simulink model "MCU_Input"  (R2022b)
settings: Solver=FixedStepDiscrete  StartTime=0.0  StopTime=10.0  FixedStep=1e-4  RelTol=1e-3
values from neighbouring files (symbols this model uses):
  C_ADC_Acc1Offset_i32 = 0.0    [MCU_Input_Sldd.sldd]    (also in MCU_Input_Sldd_objects.m = myPackage.Parameter)
  C_ADC_BrakeOffset_i32 = 0.0    [MCU_Input_Sldd.sldd]    (also in MCU_Input_Sldd_objects.m = myPackage.Parameter)
  C_ADC_HSTempGain_f32 = 0.0    [MCU_Input_Sldd.sldd]    (also in MCU_Input_Sldd_objects.m = myPackage.Parameter)
  C_ADC_HSTempOffset_i32 = 0.0    [MCU_Input_Sldd.sldd]    (also in MCU_Input_Sldd_objects.m = myPackage.Parameter)
  C_ADC_IdcOffset_i32 = 0.0    [MCU_Input_Sldd.sldd]    (also in MCU_Input_Sldd_objects.m = myPackage.Parameter)
  C_ADC_IGBTTable_i16 = 0.0    [MCU_Input_Sldd.sldd]    (also in MCU_Input_Sldd_objects.m = myPackage.Parameter)
  C_ADC_IGBTTempGain_f32 = 0.0    [MCU_Input_Sldd.sldd]    (also in MCU_Input_Sldd_objects.m = myPackage.Parameter)
  C_ADC_IGBTTempOffset_i32 = 0.0    [MCU_Input_Sldd.sldd]    (also in MCU_Input_Sldd_objects.m = myPackage.Parameter)
  C_ADC_MotorTemp1Gain_f32 = 0.0    [MCU_Input_Sldd.sldd]    (also in MCU_Input_Sldd_objects.m = myPackage.Parameter)
  C_ADC_MotorTemp1Offset_i32 = 0.0    [MCU_Input_Sldd.sldd]    (also in MCU_Input_Sldd_objects.m = myPackage.Parameter)
  C_ADC_MotorTempTable_i16 = 0.0    [MCU_Input_Sldd.sldd]    (also in MCU_Input_Sldd_objects.m = myPackage.Parameter)
  C_ADC_P12VOffset_i32 = 0.0    [MCU_Input_Sldd.sldd]    (also in MCU_Input_Sldd_objects.m = myPackage.Parameter)
  C_ADC_P15VOffset_i32 = 0.0    [MCU_Input_Sldd.sldd]    (also in MCU_Input_Sldd_objects.m = myPackage.Parameter)
  C_ADC_P5VOffset_i32 = 0.0    [MCU_Input_Sldd.sldd]    (also in MCU_Input_Sldd_objects.m = myPackage.Parameter)
  C_DCCurrent_DrvCoeff_f32 = 0.0    [MCU_Input_Sldd.sldd]    (also in MCU_Input_Sldd_objects.m = myPackage.Parameter)
  C_DCCurrent_GenCoeff_f32 = 0.0    [MCU_Input_Sldd.sldd]    (also in MCU_Input_Sldd_objects.m = myPackage.Parameter)
  C_Encoder_CurrentAdder_f32 = 0.0    [MCU_Input_Sldd.sldd]    (also in MCU_Input_Sldd_objects.m = myPackage.Parameter)
  C_Encoder_WaitTime_f32 = 0.0    [MCU_Input_Sldd.sldd]    (also in MCU_Input_Sldd_objects.m = myPackage.Parameter)
  C_Input_EncErr_u8 = 0.0    [MCU_Input_Sldd.sldd]    (also in MCU_Input_Sldd_objects.m = myPackage.Parameter)
  C_Rotate_RotateBits_u8 = 0.0    [MCU_Input_Sldd.sldd]    (also in MCU_Input_Sldd_objects.m = myPackage.Parameter)
  C_Rotate_SetAngle_u16 = 0.0    [MCU_Input_Sldd.sldd]    (also in MCU_Input_Sldd_objects.m = myPackage.Parameter)
  C_Rotate_SetAngleFlg_u8 = 0.0    [MCU_Input_Sldd.sldd]    (also in MCU_Input_Sldd_objects.m = myPackage.Parameter)
  C_SelfCheck_AvgCntSet_u16 = 0.0    [MCU_Input_Sldd.sldd]    (also in MCU_Input_Sldd_objects.m = myPackage.Parameter)
  C_SelfCheck_DelayTimeSet_u16 = 0.0    [MCU_Input_Sldd.sldd]    (also in MCU_Input_Sldd_objects.m = myPackage.Parameter)
  C_SelfCheck_IaoffsetDownLimt_u16 = 0.0    [MCU_Input_Sldd.sldd]    (also in MCU_Input_Sldd_objects.m = myPackage.Parameter)
  C_SelfCheck_IaoffsetUpLimt_u16 = 0.0    [MCU_Input_Sldd.sldd]    (also in MCU_Input_Sldd_objects.m = myPackage.Parameter)
  C_SelfCheck_IboffsetDownLimt_u16 = 0.0    [MCU_Input_Sldd.sldd]    (also in MCU_Input_Sldd_objects.m = myPackage.Parameter)
  C_SelfCheck_IboffsetUpLimt_u16 = 0.0    [MCU_Input_Sldd.sldd]    (also in MCU_Input_Sldd_objects.m = myPackage.Parameter)
  C_SelfCheck_IcoffsetDownLimt_u16 = 0.0    [MCU_Input_Sldd.sldd]    (also in MCU_Input_Sldd_objects.m = myPackage.Parameter)
  C_SelfCheck_IcoffsetUpLimt_u16 = 0.0    [MCU_Input_Sldd.sldd]    (also in MCU_Input_Sldd_objects.m = myPackage.Parameter)
  C_SelfCheck_OffsetUnCal_u8 = 0.0    [MCU_Input_Sldd.sldd]    (also in MCU_Input_Sldd_objects.m = myPackage.Parameter)
undefined symbols (not defined in the file or in its folder): AB_SAMPLE, ABC_SAMPLE, AC_SAMPLE, ANALOG, BC_SAMPLE, cAgeingMode, cParaRecogMode, cVvvfOpenMode, ParamCfg_AdAcc1K_u16, ParamCfg_AdBrakeK_u16, ParamCfg_AdIaK_u16, ParamCfg_AdIbK_u16, ParamCfg_AdIcK_u16, ParamCfg_AdKeyK_u16, ParamCfg_AdP12vK_u16, ParamCfg_AdP15vK_u16, ParamCfg_AdP5vK_u16, ParamCfg_AdUdcK_u16, ParamCfg_AdVonK_u16, ParamCfg_Avgcnt_u16, ParamCfg_BaseCur_u16, ParamCfg_BaseUdc_u16, ParamCfg_CommandSource_u16, ParamCfg_MaxSpeed_u16, ParamCfg_MotorNp_u16, ParamCfg_PosInit_u16, ParamCfg_PowerMax_u16, ParamCfg_PwmFreqLow_u16, ParamCfg_RotateDir_u16, ParamCfg_RotateNp_u16, ParamCfg_SampleMode_u16, ParamCfg_SensorSpeed_u16, ParamCfg_SmoPllKi_u16, ParamCfg_SmoPllKp_u16, ParamCfg_Stage_u16, ParamCfg_ThetaGain_u16, ParamCfg_UdcDefValue_u16, POWER_ON, STANDBY
libraries: simulink x41, YS_UserDefined_Library x4
(part 1 of 5)
settings Model: DataDictionary=MCU_Input_Sldd.sldd  Creator=ZYH  LastModifiedBy=ZYH
settings OptimizationCC: DefaultParameterBehavior=Inlined  EnhancedBackFolding=on  PassReuseOutputArgsAs=Individual arguments  OptimizeBlockOrder=speed  DifferentSizesBufferReuse=on  OptimizationCustomize=off  EfficientTunableParamExpr=on
settings DebuggingCC: ParameterTunabilityLossMsg=error
settings SFSimCC: MATLABDynamicMemAlloc=off
settings RTWCC: Description=Embedded Coder  SystemTargetFile=ert.tlc  GenCodeOnly=on  TemplateMakefile=ert_default_tmf
settings CodeAppCC: ForceParamTrailComments=on  IgnoreCustomStorageClasses=off  OperatorAnnotations=on  SimulinkDataObjDesc=on  SFDataObjDesc=on  InsertBlockDesc=on
settings ERTTargetCC: TargetLangStandard=C99 (ISO)  GenerateSampleERTMain=on  InlinedParameterPlacement=NonHierarchical  ERTCustomFileTemplate=example_file_process.tlc

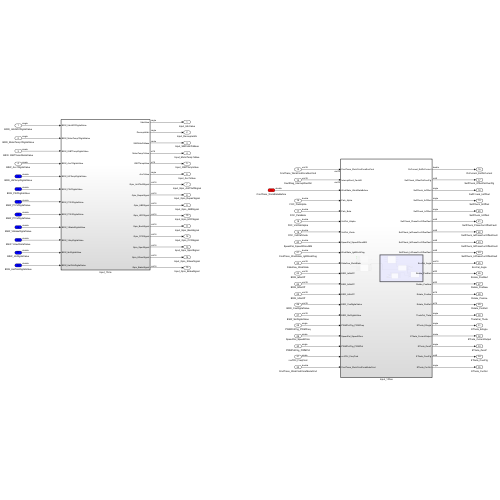
[thumbnail: Simulink's stored preview of the top-level diagram]
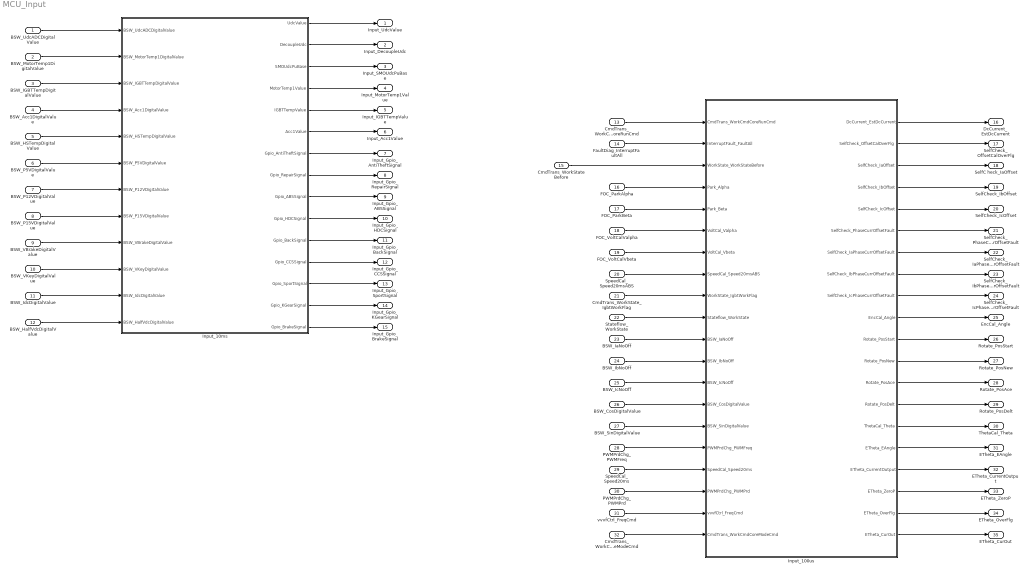
== system MCU_Input ==
  BSW_UdcADCDigitalValue : Inport
  BSW_MotorTemp1DigitalValue : Inport  Port=2
  BSW_IGBTTempDigitalValue : Inport  Port=3
  BSW_Acc1DigitalValue : Inport  Port=4
  BSW_HSTempDigitalValue : Inport  Port=5
  BSW_P5VDigitalValue : Inport  Port=6
  BSW_P12VDigitalValue : Inport  Port=7
  BSW_P15VDigitalValue : Inport  Port=8
  BSW_VBrakeDigitalValue : Inport  Port=9
  BSW_VKeyDigitalValue : Inport  Port=10
  BSW_IdcDigitalValue : Inport  Port=11
  BSW_HalfVdcDigitalValue : Inport  Port=12
  CmdTrans_WorkCmdCoreRunCmd : Inport  Port=13
  FaultDiag_InterruptFaultAll : Inport  Port=14
  CmdTrans_WorkStateBefore : Inport  Port=15
  FOC_ParkAlpha : Inport  Port=16
  FOC_ParkBeta : Inport  Port=17
  FOC_VoltCalValpha : Inport  Port=18
  FOC_VoltCalVbeta : Inport  Port=19
  SpeedCal_Speed20msABS : Inport  Port=20
  CmdTrans_WorkState_IgbtWorkFlag : Inport  Port=21
  Stateflow_WorkState : Inport  Port=22
  BSW_IaNoOff : Inport  Port=23
  BSW_IbNoOff : Inport  Port=24
  BSW_IcNoOff : Inport  Port=25
  BSW_CosDigitalValue : Inport  Port=26
  BSW_SinDigitalValue : Inport  Port=27
  PWMPrdChg_PWMFreq : Inport  Port=28
  SpeedCal_Speed20ms : Inport  Port=29
  PWMPrdChg_PWMPrd : Inport  Port=30
  vvvfCtrl_FreqCmd : Inport  Port=31
  CmdTrans_WorkCmdCoreModeCmd : Inport  Port=32
  Input_100us : Subsystem  TreatAsAtomicUnit=on
  Input_10ms : Subsystem  TreatAsAtomicUnit=on
  Input_UdcValue : Outport
  Input_DecoupleUdc : Outport  Port=2
  Input_SMOUdcPuBase : Outport  Port=3
  Input_MotorTemp1Value : Outport  Port=4
  Input_IGBTTempValue : Outport  Port=5
  Input_Acc1Value : Outport  Port=6
  Input_Gpio_AntiTheftSignal : Outport  Port=7
  Input_Gpio_RepairSignal : Outport  Port=8
  Input_Gpio_ABSSignal : Outport  Port=9
  Input_Gpio_HDCSignal : Outport  Port=10
  Input_Gpio_BackSignal : Outport  Port=11
  Input_Gpio_CCSSignal : Outport  Port=12
  Input_Gpio_SportSignal : Outport  Port=13
  Input_Gpio_KGearSignal : Outport  Port=14
  Input_Gpio_BrakeSignal : Outport  Port=15
  DcCurrent_EstDcCurrent : Outport  Port=16
  SelfCheck_OffsetCalOverFlg : Outport  Port=17
  SelfC heck_IaOffset : Outport  Port=18
  SelfCheck_IbOffset : Outport  Port=19
  SelfCheck_IcOffset : Outport  Port=20
  SelfCheck_PhaseCurrOffsetFault : Outport  Port=21
  SelfCheck_IaPhaseCurrOffsetFault : Outport  Port=22
  SelfCheck_IbPhaseCurrOffsetFault : Outport  Port=23
  SelfCheck_IcPhaseCurrOffsetFault : Outport  Port=24
  EncCal_Angle : Outport  Port=25
  Rotate_PosStart : Outport  Port=26
  Rotate_PosNew : Outport  Port=27
  Rotate_PosAce : Outport  Port=28
  Rotate_PosDelt : Outport  Port=29
  ThetaCal_Theta : Outport  Port=30
  ETheta_EAngle : Outport  Port=31
  ETheta_CurrentOutput : Outport  Port=32
  ETheta_ZeroP : Outport  Port=33
  ETheta_OverFlg : Outport  Port=34
  ETheta_CurOut : Outport  Port=35
  wires:
  BSW_IdcDigitalValue/1 -> Input_10ms/11(BSW_IdcDigitalValue)
  BSW_VKeyDigitalValue/1 -> Input_10ms/10(BSW_VKeyDigitalValue)
  Input_10ms/1(UdcValue) -> Input_UdcValue/1
  BSW_VBrakeDigitalValue/1 -> Input_10ms/9(BSW_VBrakeDigitalValue)
  BSW_P15VDigitalValue/1 -> Input_10ms/8(BSW_P15VDigitalValue)
  BSW_HalfVdcDigitalValue/1 -> Input_10ms/12(BSW_HalfVdcDigitalValue)
  BSW_Acc1DigitalValue/1 -> Input_10ms/4(BSW_Acc1DigitalValue)
  Input_10ms/5(IGBTTempValue) -> Input_IGBTTempValue/1
  Input_10ms/3(SMOUdcPuBase) -> Input_SMOUdcPuBase/1
  BSW_HSTempDigitalValue/1 -> Input_10ms/5(BSW_HSTempDigitalValue)
  BSW_P5VDigitalValue/1 -> Input_10ms/6(BSW_P5VDigitalValue)
  Input_10ms/2(DecoupleUdc) -> Input_DecoupleUdc/1
  BSW_IGBTTempDigitalValue/1 -> Input_10ms/3(BSW_IGBTTempDigitalValue)
  BSW_MotorTemp1DigitalValue/1 -> Input_10ms/2(BSW_MotorTemp1DigitalValue)
  BSW_P12VDigitalValue/1 -> Input_10ms/7(BSW_P12VDigitalValue)
  Input_10ms/6(Acc1Value) -> Input_Acc1Value/1
  Input_10ms/4(MotorTemp1Value) -> Input_MotorTemp1Value/1
  Input_10ms/7(Gpio_AntiTheftSignal) -> Input_Gpio_AntiTheftSignal/1
  Input_10ms/8(Gpio_RepairSignal) -> Input_Gpio_RepairSignal/1
  Input_10ms/9(Gpio_ABSSignal) -> Input_Gpio_ABSSignal/1
  Input_10ms/10(Gpio_HDCSignal) -> Input_Gpio_HDCSignal/1
  Input_10ms/11(Gpio_BackSignal) -> Input_Gpio_BackSignal/1
  Input_10ms/12(Gpio_CCSSignal) -> Input_Gpio_CCSSignal/1
  Input_10ms/13(Gpio_SportSignal) -> Input_Gpio_SportSignal/1
  Input_10ms/14(Gpio_KGearSignal) -> Input_Gpio_KGearSignal/1
  Input_10ms/15(Gpio_BrakeSignal) -> Input_Gpio_BrakeSignal/1
  CmdTrans_WorkCmdCoreRunCmd/1 -> Input_100us/1(CmdTrans_WorkCmdCoreRunCmd)
  FaultDiag_InterruptFaultAll/1 -> Input_100us/2(InterruptFault_FaultAll)
  Input_100us/1(DcCurrent_EstDcCurrent) -> DcCurrent_EstDcCurrent/1
  CmdTrans_WorkStateBefore/1 -> Input_100us/3(WorkState_WorkStateBefore)
  FOC_ParkAlpha/1 -> Input_100us/4(Park_Alpha)
  FOC_ParkBeta/1 -> Input_100us/5(Park_Beta)
  FOC_VoltCalValpha/1 -> Input_100us/6(VoltCal_Valpha)
  FOC_VoltCalVbeta/1 -> Input_100us/7(VoltCal_Vbeta)
  SpeedCal_Speed20msABS/1 -> Input_100us/8(SpeedCal_Speed20msABS)
  Stateflow_WorkState/1 -> Input_100us/10(Stateflow_WorkState)
  BSW_IaNoOff/1 -> Input_100us/11(BSW_IaNoOff)
  BSW_IbNoOff/1 -> Input_100us/12(BSW_IbNoOff)
  CmdTrans_WorkState_IgbtWorkFlag/1 -> Input_100us/9(WorkState_IgbtWorkFlag)
  BSW_IcNoOff/1 -> Input_100us/13(BSW_IcNoOff)
  Input_100us/3(SelfCheck_IaOffset) -> SelfC heck_IaOffset/1
  Input_100us/2(SelfCheck_OffsetCalOverFlg) -> SelfCheck_OffsetCalOverFlg/1
  Input_100us/4(SelfCheck_IbOffset) -> SelfCheck_IbOffset/1
  Input_100us/5(SelfCheck_IcOffset) -> SelfCheck_IcOffset/1
  Input_100us/6(SelfCheck_PhaseCurrOffsetFault) -> SelfCheck_PhaseCurrOffsetFault/1
  Input_100us/7(SelfCheck_IaPhaseCurrOffsetFault) -> SelfCheck_IaPhaseCurrOffsetFault/1
  Input_100us/8(SelfCheck_IbPhaseCurrOffsetFault) -> SelfCheck_IbPhaseCurrOffsetFault/1
  Input_100us/9(SelfCheck_IcPhaseCurrOffsetFault) -> SelfCheck_IcPhaseCurrOffsetFault/1
  BSW_UdcADCDigitalValue/1 -> Input_10ms/1(BSW_UdcADCDigitalValue)
  BSW_CosDigitalValue/1 -> Input_100us/14(BSW_CosDigitalValue)
  BSW_SinDigitalValue/1 -> Input_100us/15(BSW_SinDigitalValue)
  Input_100us/10(EncCal_Angle) -> EncCal_Angle/1
  Input_100us/11(Rotate_PosStart) -> Rotate_PosStart/1
  Input_100us/12(Rotate_PosNew) -> Rotate_PosNew/1
  Input_100us/13(Rotate_PosAce) -> Rotate_PosAce/1
  Input_100us/14(Rotate_PosDelt) -> Rotate_PosDelt/1
  SpeedCal_Speed20ms/1 -> Input_100us/17(SpeedCal_Speed20ms)
  PWMPrdChg_PWMPrd/1 -> Input_100us/18(PWMPrdChg_PWMPrd)
  vvvfCtrl_FreqCmd/1 -> Input_100us/19(vvvfCtrl_FreqCmd)
  CmdTrans_WorkCmdCoreModeCmd/1 -> Input_100us/20(CmdTrans_WorkCmdCoreModeCmd)
  Input_100us/15(ThetaCal_Theta) -> ThetaCal_Theta/1
  Input_100us/16(ETheta_EAngle) -> ETheta_EAngle/1
  Input_100us/17(ETheta_CurrentOutput) -> ETheta_CurrentOutput/1
  Input_100us/18(ETheta_ZeroP) -> ETheta_ZeroP/1
  Input_100us/19(ETheta_OverFlg) -> ETheta_OverFlg/1
  Input_100us/20(ETheta_CurOut) -> ETheta_CurOut/1
  PWMPrdChg_PWMFreq/1 -> Input_100us/16(PWMPrdChg_PWMFreq)

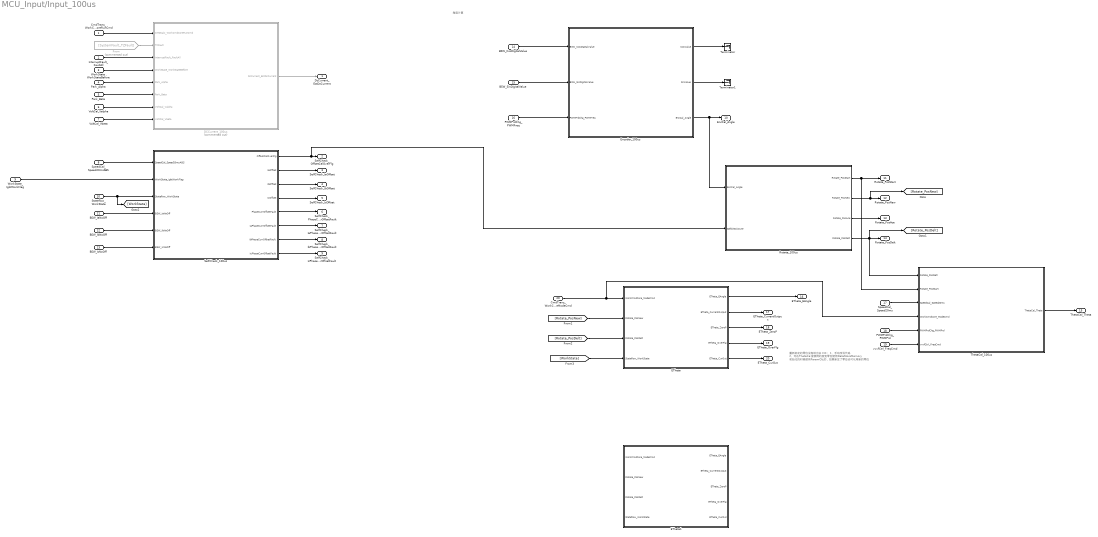
== system MCU_Input/Input_100us ==
  note: 重新标定的零位没有给出去
      | FIX：
      | 1、手动改写代码
      | 2、对在ThetaCal里使用的旋变零位使用DataStoreMemory
      | 	初始化的时候使用ParamCfg的，如果新定了零位也可以用新的零位
  note: 角度计算
  CmdTrans_WorkCmdCoreRunCmd : Inport  OutDataTypeStr=uint16
  InterruptFault_FaultAll : Inport  Port=2  OutDataTypeStr=uint16
  WorkState_WorkStateBefore : Inport  Port=3
  Park_Alpha : Inport  Port=4
  Park_Beta : Inport  Port=5
  VoltCal_Valpha : Inport  Port=6
  VoltCal_Vbeta : Inport  Port=7
  SpeedCal_Speed20msABS : Inport  Port=8
  WorkState_IgbtWorkFlag : Inport  Port=9
  Stateflow_WorkState : Inport  Port=10
  BSW_IaNoOff : Inport  Port=11
  BSW_IbNoOff : Inport  Port=12
  BSW_IcNoOff : Inport  Port=13
  BSW_CosDigitalValue : Inport  Port=14
  BSW_SinDigitalValue : Inport  Port=15
  PWMPrdChg_PWMFreq : Inport  Port=16
  SpeedCal_Speed20ms : Inport  Port=17
  PWMPrdChg_PWMPrd : Inport  Port=18
  vvvfCtrl_FreqCmd : Inport  Port=19
  CmdTrans_WorkCmdCoreModeCmd : Inport  Port=20
  DCCurrent_100us : Subsystem  Commented=on  TreatAsAtomicUnit=on
      settings: RTWSystemCode=Nonreusable function
  ETheta : Subsystem
  ETheta1 : Subsystem
  Encoder_100us : Subsystem  TreatAsAtomicUnit=on
      settings: RTWSystemCode=Nonreusable function
  From : From  Commented=on  GotoTag=SystemFault_TZFault
  Rotate_100us : Subsystem  TreatAsAtomicUnit=on
      settings: RTWSystemCode=Nonreusable function
  SelfCheck_100us : Subsystem  TreatAsAtomicUnit=on
      settings: RTWSystemCode=Nonreusable function
  Terminator : Terminator
  Terminator1 : Terminator
  ThetaCal_100us : Subsystem
  DcCurrent_EstDcCurrent : Outport
  SelfCheck_OffsetCalOverFlg : Outport  Port=2
  SelfCheck_IaOffset : Outport  Port=3
  SelfCheck_IbOffset : Outport  Port=4
  SelfCheck_IcOffset : Outport  Port=5
  SelfCheck_PhaseCurrOffsetFault : Outport  Port=6
  SelfCheck_IaPhaseCurrOffsetFault : Outport  Port=7
  SelfCheck_IbPhaseCurrOffsetFault : Outport  Port=8
  SelfCheck_IcPhaseCurrOffsetFault : Outport  Port=9
  EncCal_Angle : Outport  Port=10
  Rotate_PosStart : Outport  Port=11
  Rotate_PosNew : Outport  Port=12
  Rotate_PosAce : Outport  Port=13
  Rotate_PosDelt : Outport  Port=14
  ThetaCal_Theta : Outport  Port=15
  ETheta_EAngle : Outport  Port=16
  ETheta_CurrentOutput : Outport  Port=17
  ETheta_ZeroP : Outport  Port=18
  ETheta_OverFlg : Outport  Port=19
  ETheta_CurOut : Outport  Port=20
  wires:
  CmdTrans_WorkCmdCoreRunCmd/1 -> DCCurrent_100us/1(CMDCalc_WorkCmdCoreRunCmd)
  From/1 -> DCCurrent_100us/2(TZFault)
  InterruptFault_FaultAll/1 -> DCCurrent_100us/3(InterruptFault_FaultAll)
  DCCurrent_100us/1(DcCurrent_EstDcCurrent) -> DcCurrent_EstDcCurrent/1
  WorkState_WorkStateBefore/1 -> DCCurrent_100us/4(WorkState_WorkStateBefore)
  Park_Alpha/1 -> DCCurrent_100us/5(Park_Alpha)
  Park_Beta/1 -> DCCurrent_100us/6(Park_Beta)
  VoltCal_Valpha/1 -> DCCurrent_100us/7(VoltCal_Valpha)
  VoltCal_Vbeta/1 -> DCCurrent_100us/8(VoltCal_Vbeta)
  SpeedCal_Speed20msABS/1 -> SelfCheck_100us/1(SpeedCal_Speed20msABS)
  WorkState_IgbtWorkFlag/1 -> SelfCheck_100us/2(WorkState_IgbtWorkFlag)
  Stateflow_WorkState/1 -> [WorkState], SelfCheck_100us/3(Stateflow_WorkState)
  BSW_IaNoOff/1 -> SelfCheck_100us/4(BSW_IaNoOff)
  BSW_IbNoOff/1 -> SelfCheck_100us/5(BSW_IbNoOff)
  BSW_IcNoOff/1 -> SelfCheck_100us/6(BSW_IcNoOff)
  SelfCheck_100us/1(OffsetCalOverFlg) -> Rotate_100us/2(SelfCheckOver), SelfCheck_OffsetCalOverFlg/1
  SelfCheck_100us/2(IaOffset) -> SelfCheck_IaOffset/1
  SelfCheck_100us/5(PhaseCurrOffsetFault) -> SelfCheck_PhaseCurrOffsetFault/1
  SelfCheck_100us/4(IcOffset) -> SelfCheck_IcOffset/1
  SelfCheck_100us/3(IbOffset) -> SelfCheck_IbOffset/1
  SelfCheck_100us/7(IbPhaseCurrOffsetFault) -> SelfCheck_IbPhaseCurrOffsetFault/1
  SelfCheck_100us/6(IaPhaseCurrOffsetFault) -> SelfCheck_IaPhaseCurrOffsetFault/1
  SelfCheck_100us/8(IcPhaseCurrOffsetFault) -> SelfCheck_IcPhaseCurrOffsetFault/1
  BSW_CosDigitalValue/1 -> Encoder_100us/1(BSW_CosDigitalValue)
  BSW_SinDigitalValue/1 -> Encoder_100us/2(BSW_SinDigitalValue)
  Encoder_100us/1(CosValue) -> Terminator/1
  Encoder_100us/2(SinValue) -> Terminator1/1
  Encoder_100us/3(EncCal_Angle) -> Rotate_100us/1(EncCal_Angle), EncCal_Angle/1
  Rotate_100us/1(Rotate_PosStart) -> ThetaCal_100us/2(Rotate_PosStart), Rotate_PosStart/1
  Rotate_100us/2(Rotate_PosNew) -> [Rotate_PosNew], Rotate_PosNew/1
  Rotate_100us/3(Rotate_PosAce) -> Rotate_PosAce/1
  Rotate_100us/4(Rotate_PosDelt) -> ThetaCal_100us/1(Rotate_PosDelt), [Rotate_PosDelt], Rotate_PosDelt/1
  SpeedCal_Speed20ms/1 -> ThetaCal_100us/3(SpeedCal_Speed20ms)
  ThetaCal_100us/1(ThetaCal_Theta) -> ThetaCal_Theta/1
  CmdTrans_WorkCmdCoreModeCmd/1 -> ThetaCal_100us/4(WorkCmdCore_ModeCmd), ETheta/1(WorkCmdCore_ModeCmd)
  PWMPrdChg_PWMPrd/1 -> ThetaCal_100us/5(PWMPrdChg_PWMPrd)
  vvvfCtrl_FreqCmd/1 -> ThetaCal_100us/6(vvvfCtrl_FreqCmd)
  [Rotate_PosNew] -> ETheta/2(Rotate_PosNew)
  [Rotate_PosDelt] -> ETheta/3(Rotate_PosDelt)
  ETheta/1(ETheta_EAngle) -> ETheta_EAngle/1
  ETheta/2(ETheta_CurrentOutput) -> ETheta_CurrentOutput/1
  ETheta/3(ETheta_ZeroP) -> ETheta_ZeroP/1
  ETheta/4(ETheta_OverFlg) -> ETheta_OverFlg/1
  ETheta/5(ETheta_CurOut) -> ETheta_CurOut/1
  PWMPrdChg_PWMFreq/1 -> Encoder_100us/3(PWMPrdChg_PWMFreq)
  [WorkState] -> ETheta/4(Stateflow_WorkState)

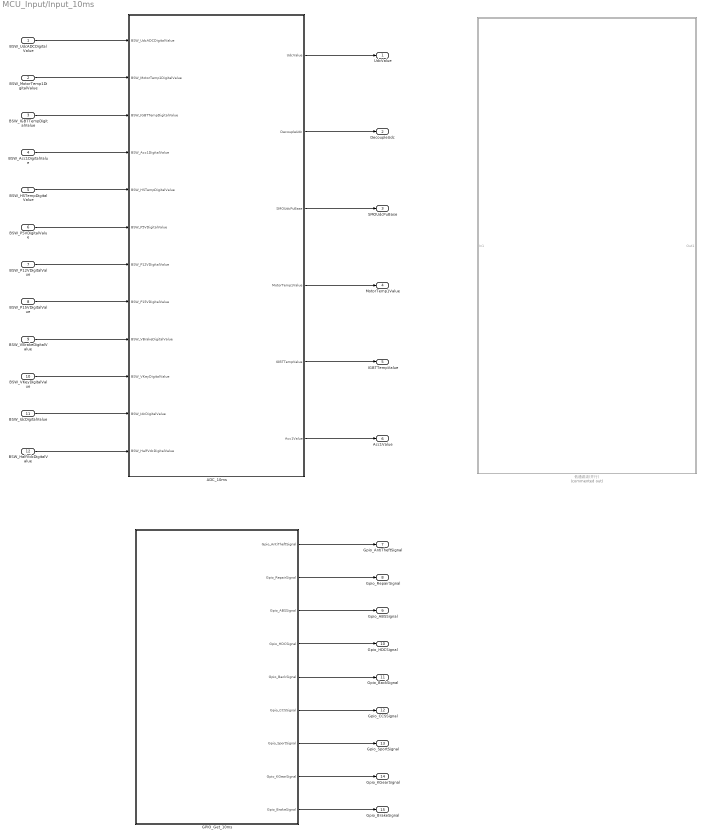
== system MCU_Input/Input_10ms ==
  BSW_UdcADCDigitalValue : Inport
  BSW_MotorTemp1DigitalValue : Inport  Port=2
  BSW_IGBTTempDigitalValue : Inport  Port=3
  BSW_Acc1DigitalValue : Inport  Port=4
  BSW_HSTempDigitalValue : Inport  Port=5
  BSW_P5VDigitalValue : Inport  Port=6
  BSW_P12VDigitalValue : Inport  Port=7
  BSW_P15VDigitalValue : Inport  Port=8
  BSW_VBrakeDigitalValue : Inport  Port=9
  BSW_VKeyDigitalValue : Inport  Port=10
  BSW_IdcDigitalValue : Inport  Port=11
  BSW_HalfVdcDigitalValue : Inport  Port=12
  ADC_10ms : Subsystem  TreatAsAtomicUnit=on
      settings: RTWSystemCode=Nonreusable function
  GPIO_Get_10ms : Subsystem  TreatAsAtomicUnit=on
      settings: RTWSystemCode=Nonreusable function
  低通滤波(并行) : Subsystem  Commented=on
  UdcValue : Outport
  DecoupleUdc : Outport  Port=2
  SMOUdcPuBase : Outport  Port=3
  MotorTemp1Value : Outport  Port=4
  IGBTTempValue : Outport  Port=5
  Acc1Value : Outport  Port=6
  Gpio_AntiTheftSignal : Outport  Port=7
  Gpio_RepairSignal : Outport  Port=8
  Gpio_ABSSignal : Outport  Port=9
  Gpio_HDCSignal : Outport  Port=10
  Gpio_BackSignal : Outport  Port=11
  Gpio_CCSSignal : Outport  Port=12
  Gpio_SportSignal : Outport  Port=13
  Gpio_KGearSignal : Outport  Port=14
  Gpio_BrakeSignal : Outport  Port=15
  wires:
  BSW_MotorTemp1DigitalValue/1 -> ADC_10ms/2(BSW_MotorTemp1DigitalValue)
  BSW_IGBTTempDigitalValue/1 -> ADC_10ms/3(BSW_IGBTTempDigitalValue)
  BSW_Acc1DigitalValue/1 -> ADC_10ms/4(BSW_Acc1DigitalValue)
  BSW_HSTempDigitalValue/1 -> ADC_10ms/5(BSW_HSTempDigitalValue)
  BSW_P5VDigitalValue/1 -> ADC_10ms/6(BSW_P5VDigitalValue)
  BSW_P12VDigitalValue/1 -> ADC_10ms/7(BSW_P12VDigitalValue)
  BSW_P15VDigitalValue/1 -> ADC_10ms/8(BSW_P15VDigitalValue)
  BSW_VBrakeDigitalValue/1 -> ADC_10ms/9(BSW_VBrakeDigitalValue)
  BSW_VKeyDigitalValue/1 -> ADC_10ms/10(BSW_VKeyDigitalValue)
  BSW_IdcDigitalValue/1 -> ADC_10ms/11(BSW_IdcDigitalValue)
  BSW_HalfVdcDigitalValue/1 -> ADC_10ms/12(BSW_HalfVdcDigitalValue)
  ADC_10ms/4(MotorTemp1Value) -> MotorTemp1Value/1
  ADC_10ms/3(SMOUdcPuBase) -> SMOUdcPuBase/1
  ADC_10ms/5(IGBTTempValue) -> IGBTTempValue/1
  ADC_10ms/2(DecoupleUdc) -> DecoupleUdc/1
  ADC_10ms/6(Acc1Value) -> Acc1Value/1
  ADC_10ms/1(UdcValue) -> UdcValue/1
  GPIO_Get_10ms/1(Gpio_AntiTheftSignal) -> Gpio_AntiTheftSignal/1
  GPIO_Get_10ms/2(Gpio_RepairSignal) -> Gpio_RepairSignal/1
  GPIO_Get_10ms/3(Gpio_ABSSignal) -> Gpio_ABSSignal/1
  GPIO_Get_10ms/4(Gpio_HDCSignal) -> Gpio_HDCSignal/1
  GPIO_Get_10ms/5(Gpio_BackSignal) -> Gpio_BackSignal/1
  GPIO_Get_10ms/6(Gpio_CCSSignal) -> Gpio_CCSSignal/1
  GPIO_Get_10ms/7(Gpio_SportSignal) -> Gpio_SportSignal/1
  GPIO_Get_10ms/8(Gpio_KGearSignal) -> Gpio_KGearSignal/1
  GPIO_Get_10ms/9(Gpio_BrakeSignal) -> Gpio_BrakeSignal/1
  BSW_UdcADCDigitalValue/1 -> ADC_10ms/1(BSW_UdcADCDigitalValue)

== system MCU_Input/Input_100us/DCCurrent_100us ==
  CMDCalc_WorkCmdCoreRunCmd : Inport
  TZFault : Inport  Port=2
  InterruptFault_FaultAll : Inport  Port=3
  WorkState_WorkStateBefore : Inport  Port=4
  Park_Alpha : Inport  Port=5
  Park_Beta : Inport  Port=6
  VoltCal_Valpha : Inport  Port=7
  VoltCal_Vbeta : Inport  Port=8
  Compare To Constant : simulink/Logic and Bit Operations/Compare To Constant  relop===  const=1  OutDataTypeStr=boolean
  Compare To Constant1 : simulink/Logic and Bit Operations/Compare To Constant  relop===  const=0  OutDataTypeStr=boolean
  Compare To Constant2 : simulink/Logic and Bit Operations/Compare To Constant  relop===  const=0  OutDataTypeStr=boolean
  DcCurrentCal : Subsystem  TreatAsAtomicUnit=on
  Logical Operator : Logic  Inputs=3  AllPortsSameDT=off  OutDataTypeStr=boolean
  DcCurrent_EstDcCurrent : Outport
  wires:
  CMDCalc_WorkCmdCoreRunCmd/1 -> Compare To Constant/1
  TZFault/1 -> Compare To Constant1/1
  InterruptFault_FaultAll/1 -> Compare To Constant2/1
  Compare To Constant1/1 -> Logical Operator/2
  Compare To Constant2/1 -> Logical Operator/3
  Compare To Constant/1 -> Logical Operator/1
  Logical Operator/1 -> DcCurrentCal/Enable
  DcCurrentCal/1(DcCurrent_EstDcCurrent) -> DcCurrent_EstDcCurrent/1
  WorkState_WorkStateBefore/1 -> DcCurrentCal/1(WorkState_WorkStateBefore)
  Park_Alpha/1 -> DcCurrentCal/2(Park_Alpha)
  Park_Beta/1 -> DcCurrentCal/3(Park_Beta)
  VoltCal_Valpha/1 -> DcCurrentCal/4(VoltCal_Valpha)
  VoltCal_Vbeta/1 -> DcCurrentCal/5(VoltCal_Vbeta)

== system MCU_Input/Input_100us/ETheta ==
  WorkCmdCore_ModeCmd : Inport
  Rotate_PosNew : Inport  Port=2
  Rotate_PosDelt : Inport  Port=3
  Stateflow_WorkState : Inport  Port=4
  Compare To Constant : simulink/Logic and Bit Operations/Compare To Constant  relop===  const=cParaRecogMode  OutDataTypeStr=boolean
  Compare To Constant1 : simulink/Logic and Bit Operations/Compare To Constant  relop===  const=STANDBY  OutDataTypeStr=boolean
  Constant : Constant  Value=0  OutDataTypeStr=single
  En : Subsystem
  Switch : Switch  Criteria=u2 ~= 0  SaturateOnIntegerOverflow=off  InputSameDT=off
  Switch1 : Switch  Criteria=u2 ~= 0  SaturateOnIntegerOverflow=off  InputSameDT=off
  ETheta_EAngle : Outport
  ETheta_CurrentOutput : Outport  Port=2
  ETheta_ZeroP : Outport  Port=3
  ETheta_OverFlg : Outport  Port=4
  ETheta_CurOut : Outport  Port=5
  wires:
  Rotate_PosNew/1 -> En/1(Rotate_PosNew)
  Rotate_PosDelt/1 -> En/2(Rotate_PosDelt)
  WorkCmdCore_ModeCmd/1 -> Compare To Constant/1
  Compare To Constant/1 -> En/Enable
  En/1(EAngle) -> Switch/3
  En/2(CurrentOutput) -> Switch1/3
  En/4(OverFlg) -> ?
  En/5(CurOut) -> ?
  Stateflow_WorkState/1 -> Compare To Constant1/1
  Compare To Constant1/1 -> Switch1/2, Switch/2
  Constant/1 -> Switch1/1, Switch/1
  Switch/1 -> ETheta_EAngle/1
  Switch1/1 -> ETheta_CurrentOutput/1
  En/3(ZeroP) -> ETheta_ZeroP/1

== system MCU_Input/Input_100us/ETheta1 ==
  WorkCmdCore_ModeCmd : Inport
  Rotate_PosNew : Inport  Port=2
  Rotate_PosDelt : Inport  Port=3
  Stateflow_WorkState : Inport  Port=4
  Compare To Constant : simulink/Logic and Bit Operations/Compare To Constant  relop===  const=cParaRecogMode  OutDataTypeStr=boolean
  Compare To Constant1 : simulink/Logic and Bit Operations/Compare To Constant  relop===  const=STANDBY  OutDataTypeStr=boolean
  En : Subsystem
  ETheta_EAngle : Outport
  ETheta_CurrentOutput : Outport  Port=2
  ETheta_ZeroP : Outport  Port=3
  ETheta_OverFlg : Outport  Port=4
  ETheta_CurOut : Outport  Port=5
  wires:
  Rotate_PosNew/1 -> En/2(Rotate_PosNew)
  Rotate_PosDelt/1 -> En/3(Rotate_PosDelt)
  WorkCmdCore_ModeCmd/1 -> Compare To Constant/1
  Compare To Constant/1 -> En/1(cParaRecogMode)
  Stateflow_WorkState/1 -> Compare To Constant1/1
  Compare To Constant1/1 -> En/4(Standby)
  En/3(ZeroP) -> ETheta_ZeroP/1
  En/1(EAngle) -> ETheta_EAngle/1
  En/2(CurrentOutput) -> ETheta_CurrentOutput/1
  En/4(OverFlg) -> ETheta_OverFlg/1
  En/5(CurOut) -> ETheta_CurOut/1

== system MCU_Input/Input_100us/Encoder_100us ==
  note: 源代码这里除了有感还有无感，才有了这个使能，模型现在只有有感，暂时屏蔽这个使能
  BSW_CosDigitalValue : Inport
  BSW_SinDigitalValue : Inport  Port=2
  PWMPrdChg_PWMFreq : Inport  Port=3
  Compare To Constant : simulink/Logic and Bit Operations/Compare To Constant  Commented=on  relop===  const=1  OutDataTypeStr=boolean
  Constant : Constant  Value=ParamCfg_Stage_u16
  Constant1 : Constant  Value=ParamCfg_Avgcnt_u16
  Constant2 : Constant  Commented=on  Value=ParamCfg_SensorSpeed_u16
  Encoder_100us : Subsystem
  CosValue : Outport
  SinValue : Outport  Port=2
  EncCal_Angle : Outport  Port=3
  wires:
  BSW_CosDigitalValue/1 -> Encoder_100us/3(CosDigitalValue)
  BSW_SinDigitalValue/1 -> Encoder_100us/4(SinDigitalValue)
  Encoder_100us/1(CosAverage) -> CosValue/1
  Encoder_100us/2(SinAverage) -> SinValue/1
  Constant/1 -> Encoder_100us/1(Calib_Stage)
  Constant1/1 -> Encoder_100us/2(AvgCnt)
  Encoder_100us/3(EncCal_Angle) -> EncCal_Angle/1
  PWMPrdChg_PWMFreq/1 -> Encoder_100us/5(PWMPrdChg_PWMFreq)
  Constant2/1 -> Compare To Constant/1

== system MCU_Input/Input_100us/Rotate_100us ==
  EncCal_Angle : Inport
  SelfCheckOver : Inport  Port=2
  RotateCalc : Subsystem
  Rotate_PosStart : Outport
  Rotate_PosNew : Outport  Port=2
  Rotate_PosAce : Outport  Port=3
  Rotate_PosDelt : Outport  Port=4
  wires:
  EncCal_Angle/1 -> RotateCalc/1(EncCal_Angle)
  RotateCalc/1(Rotate_PosStart) -> Rotate_PosStart/1
  RotateCalc/2(Rotate_PosNew) -> Rotate_PosNew/1
  RotateCalc/3(Rotate_PosAce) -> Rotate_PosAce/1
  RotateCalc/4(Rotate_PosDelt) -> Rotate_PosDelt/1
  SelfCheckOver/1 -> RotateCalc/2(SelfCheckOver)

== system MCU_Input/Input_100us/SelfCheck_100us ==
  note: 在standby状态下持续执行
      | 在poweron状态下只执行一次
  SpeedCal_Speed20msABS : Inport
  WorkState_IgbtWorkFlag : Inport  Port=2
  Stateflow_WorkState : Inport  Port=3  OutDataTypeStr=uint16
  BSW_IaNoOff : Inport  Port=4
  BSW_IbNoOff : Inport  Port=5
  BSW_IcNoOff : Inport  Port=6
  Compare To Constant : simulink/Logic and Bit Operations/Compare To Constant  relop===  const=POWER_ON  OutDataTypeStr=uint8
  Compare To Constant2 : simulink/Logic and Bit Operations/Compare To Constant  relop===  const=STANDBY  OutDataTypeStr=uint8
  Constant : Constant  Value=C_SelfCheck_DelayTimeSet_u16  OutDataTypeStr=uint16
  Constant1 : Constant  Value=C_SelfCheck_AvgCntSet_u16  OutDataTypeStr=uint16
  Constant4 : Constant  Value=ParamCfg_SampleMode_u16
  EnCal : Subsystem
  OffsetCal : Subsystem
      settings: RTWSystemCode=Inline
  OffsetCalOverFlg : Outport
  IaOffset : Outport  Port=2
  IbOffset : Outport  Port=3
  IcOffset : Outport  Port=4
  PhaseCurrOffsetFault : Outport  Port=5
  IaPhaseCurrOffsetFault : Outport  Port=6
  IbPhaseCurrOffsetFault : Outport  Port=7
  IcPhaseCurrOffsetFault : Outport  Port=8
  wires:
  Constant4/1 -> OffsetCal/3(ParamCfg_SampleMode)
  OffsetCal/4(IcOffset) -> IcOffset/1
  Compare To Constant2/1 -> OffsetCal/1(StandbyState), EnCal/3(StanbyState)
  Constant1/1 -> OffsetCal/8(AvgCntSet)
  Compare To Constant/1 -> OffsetCal/2(PoweronState), EnCal/4(PoweronState)
  OffsetCal/7(IbOffsetFault) -> IbPhaseCurrOffsetFault/1
  OffsetCal/1(OffsetCalOverFlg) -> [OffsetCalOverFlg], OffsetCalOverFlg/1
  OffsetCal/3(IbOffset) -> IbOffset/1
  BSW_IcNoOff/1 -> OffsetCal/6(BSW_IcNoOff)
  OffsetCal/5(PhaseCurrOffsetFault) -> PhaseCurrOffsetFault/1
  Stateflow_WorkState/1 -> Compare To Constant/1, Compare To Constant2/1
  Constant/1 -> OffsetCal/7(DelayTimeSet)
  OffsetCal/8(IcOffsetFault) -> IcPhaseCurrOffsetFault/1
  OffsetCal/2(IaOffset) -> IaOffset/1
  BSW_IbNoOff/1 -> OffsetCal/5(BSW_IbNoOff)
  OffsetCal/6(IaOffsetFault) -> IaPhaseCurrOffsetFault/1
  BSW_IaNoOff/1 -> OffsetCal/4(BSW_IaNoOff)
  SpeedCal_Speed20msABS/1 -> EnCal/1(SpeedCal_Speed20msABS)
  WorkState_IgbtWorkFlag/1 -> EnCal/2(WorkState_IgbtWorkFlag)
  EnCal/1(M_Selfcheck_EnFlg_u8) -> OffsetCal/Enable
  [OffsetCalOverFlg] -> EnCal/5(OffsetCalOverFlg)

== system MCU_Input/Input_100us/ThetaCal_100us ==
  Rotate_PosDelt : Inport
  Rotate_PosStart : Inport  Port=2
  SpeedCal_Speed20ms : Inport  Port=3
  WorkCmdCore_ModeCmd : Inport  Port=4
  PWMPrdChg_PWMPrd : Inport  Port=5
  vvvfCtrl_FreqCmd : Inport  Port=6
  Compare To Constant : simulink/Logic and Bit Operations/Compare To Constant  relop===  const=1  OutDataTypeStr=boolean
  Compare To Constant1 : simulink/Logic and Bit Operations/Compare To Constant  relop===  const=cVvvfOpenMode  OutDataTypeStr=boolean
  Compare To Constant2 : simulink/Logic and Bit Operations/Compare To Constant  relop===  const=cAgeingMode  OutDataTypeStr=boolean
  Compare To Constant3 : simulink/Logic and Bit Operations/Compare To Constant  relop=>  const=1  OutDataTypeStr=boolean
  Compare To Constant4 : simulink/Logic and Bit Operations/Compare To Constant  relop=<  const=0  OutDataTypeStr=boolean
  Constant : Constant  Value=ParamCfg_SensorSpeed_u16
  Constant4 : Constant  Value=0  OutDataTypeStr=single
  If : If  NumInputs=2  IfExpression=u1 == 1  ElseIfExpressions=u2==1
  If Action Subsystem : Subsystem  TreatAsAtomicUnit=on
  If Action Subsystem1 : Subsystem  TreatAsAtomicUnit=on
  If Action Subsystem2 : Subsystem  TreatAsAtomicUnit=on
  Logical Operator : Logic  Operator=OR  AllPortsSameDT=off  OutDataTypeStr=boolean
  Merge : Merge  Inputs=3
  Switch : Switch  Criteria=u2 ~= 0  SaturateOnIntegerOverflow=off  InputSameDT=off
  ThetaCal : Subsystem
  ThetaOffsetGain : Subsystem
  ThetaCal_Theta : Outport
  wires:
  Constant/1 -> ThetaOffsetGain/1(SpeedSensor), Compare To Constant/1
  Rotate_PosDelt/1 -> ThetaCal/1(Rotate_PosDelt)
  Rotate_PosStart/1 -> ThetaCal/2(Rotate_PosStart)
  SpeedCal_Speed20ms/1 -> ThetaOffsetGain/2(SpeedCal_Speed20ms)
  ThetaOffsetGain/1(PosCompensate) -> ThetaCal/3(PosCompensate)
  Compare To Constant/1 -> ThetaCal/Enable
  WorkCmdCore_ModeCmd/1 -> Compare To Constant2/1, Compare To Constant1/1
  Compare To Constant1/1 -> If/1
  Compare To Constant2/1 -> If/2
  If/1 -> If Action Subsystem/Action
  PWMPrdChg_PWMPrd/1 -> If Action Subsystem1/1(PWMPrdChg_PWMPrd), If Action Subsystem/1(PWMPrdChg_PWMPrd)
  vvvfCtrl_FreqCmd/1 -> If Action Subsystem1/2(vvvfCtrl_FreqCmd), If Action Subsystem/2(vvvfCtrl_FreqCmd)
  If/2 -> If Action Subsystem1/Action
  If/3 -> If Action Subsystem2/Action
  ThetaCal/1(POSTheta) -> If Action Subsystem2/1(POSTheta)
  If Action Subsystem/1(mTheta) -> Merge/1
  If Action Subsystem1/1(mTheta) -> Merge/2
  If Action Subsystem2/1(mTheta) -> Merge/3
  Merge/1 -> Switch/3, Compare To Constant4/1, Compare To Constant3/1
  Constant4/1 -> Switch/1
  Compare To Constant4/1 -> Logical Operator/2
  Compare To Constant3/1 -> Logical Operator/1
  Logical Operator/1 -> Switch/2
  Switch/1 -> ThetaCal_Theta/1

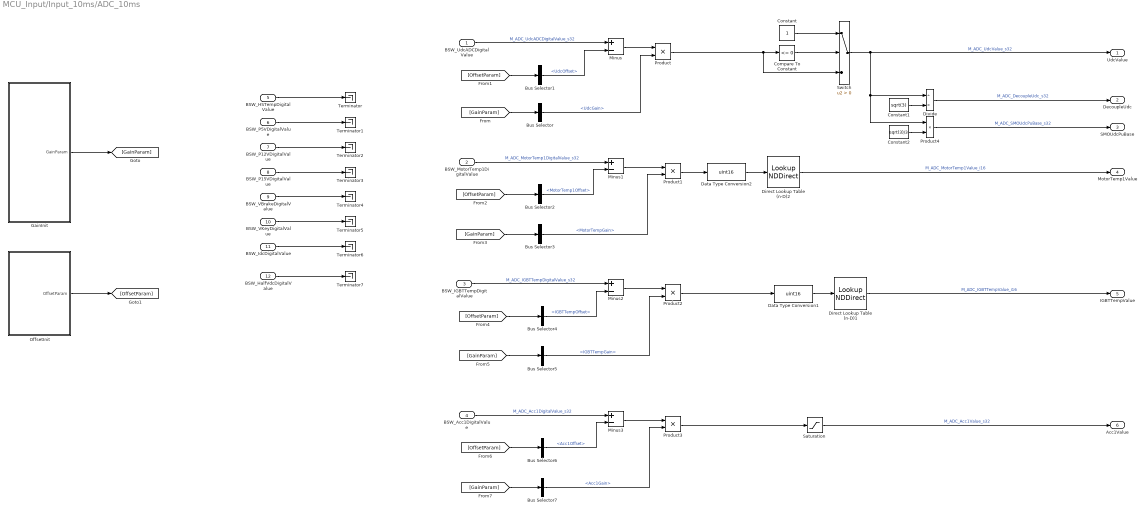
== system MCU_Input/Input_10ms/ADC_10ms ==
  BSW_UdcADCDigitalValue : Inport
  BSW_MotorTemp1DigitalValue : Inport  Port=2
  BSW_IGBTTempDigitalValue : Inport  Port=3
  BSW_Acc1DigitalValue : Inport  Port=4
  BSW_HSTempDigitalValue : Inport  Port=5
  BSW_P5VDigitalValue : Inport  Port=6
  BSW_P12VDigitalValue : Inport  Port=7
  BSW_P15VDigitalValue : Inport  Port=8
  BSW_VBrakeDigitalValue : Inport  Port=9
  BSW_VKeyDigitalValue : Inport  Port=10
  BSW_IdcDigitalValue : Inport  Port=11
  BSW_HalfVdcDigitalValue : Inport  Port=12
  Bus Selector : BusSelector  OutputSignals=UdcGain
  Bus Selector1 : BusSelector  OutputSignals=UdcOffset
  Bus Selector2 : BusSelector  OutputSignals=MotorTemp1Offset
  Bus Selector3 : BusSelector  OutputSignals=MotorTempGain
  Bus Selector4 : BusSelector  OutputSignals=IGBTTempOffset
  Bus Selector5 : BusSelector  OutputSignals=IGBTTempGain
  Bus Selector6 : BusSelector  OutputSignals=Acc1Offset
  Bus Selector7 : BusSelector  OutputSignals=Acc1Gain
  Compare To Constant : simulink/Logic and Bit Operations/Compare To Constant  relop=<=  const=0  OutDataTypeStr=boolean
  Constant : Constant  OutDataTypeStr=single
  Constant1 : Constant  Value=sqrt(3)  OutDataTypeStr=single
  Constant2 : Constant  Value=sqrt(3)/3  OutDataTypeStr=single
  Data Type Conversion1 : DataTypeConversion  OutDataTypeStr=uint16  SaturateOnIntegerOverflow=off  RndMeth=Floor
  Data Type Conversion2 : DataTypeConversion  OutDataTypeStr=uint16  SaturateOnIntegerOverflow=off  RndMeth=Floor
  Direct Lookup Table (n-D)1 : LookupNDDirect  NumberOfTableDimensions=1  Table=C_ADC_IGBTTable_i16  TableDataTypeStr=int16
  Direct Lookup Table (n-D)2 : LookupNDDirect  NumberOfTableDimensions=1  Table=C_ADC_MotorTempTable_i16  TableDataTypeStr=int16
  Divide : Product  Inputs=/*
  GainInit : Subsystem
      settings: RTWSystemCode=Nonreusable function
  Minus{,1..3} (4 alike) : Sum  Inputs=+-
  OffsetInit : Subsystem
  Product{,1..4} (5 alike) : Product
  Saturation : Saturate  UpperLimit=1  LowerLimit=0
  Switch : Switch  Criteria=u2 > Threshold  SaturateOnIntegerOverflow=off  InputSameDT=off
  Terminator{,1..7} (8 alike) : Terminator
  UdcValue : Outport
  DecoupleUdc : Outport  Port=2
  SMOUdcPuBase : Outport  Port=3
  MotorTemp1Value : Outport  Port=4
  IGBTTempValue : Outport  Port=5
  Acc1Value : Outport  Port=6
  wires:
  BSW_HalfVdcDigitalValue/1 -> Terminator7/1
  BSW_UdcADCDigitalValue/1 -> Minus/1  "M_ADC_UdcADCDigitalValue_s32"
  Divide/1 -> DecoupleUdc/1  "M_ADC_DecoupleUdc_s32"
  [GainParam] -> Bus Selector/1
  BSW_Acc1DigitalValue/1 -> Minus3/1  "M_ADC_Acc1DigitalValue_s32"
  BSW_P15VDigitalValue/1 -> Terminator3/1
  BSW_P12VDigitalValue/1 -> Terminator2/1
  Saturation/1 -> Acc1Value/1  "M_ADC_Acc1Value_s32"
  BSW_P5VDigitalValue/1 -> Terminator1/1
  BSW_IGBTTempDigitalValue/1 -> Minus2/1  "M_ADC_IGBTTempDigitalValue_s32"
  Bus Selector/1 -> Product/2  "<UdcGain>"
  Bus Selector1/1 -> Minus/2  "<UdcOffset>"
  GainInit/1(GainParam) -> [GainParam]
  Switch/1 -> Product4/1, Divide/1, UdcValue/1  "M_ADC_UdcValue_s32"
  Constant2/1 -> Product4/2
  Data Type Conversion1/1 -> Direct Lookup Table (n-D)1/1
  [OffsetParam] -> Bus Selector4/1
  Constant1/1 -> Divide/2
  Minus2/1 -> Product2/1
  Bus Selector6/1 -> Minus3/2  "<Acc1Offset>"
  BSW_MotorTemp1DigitalValue/1 -> Minus1/1  "M_ADC_MotorTemp1DigitalValue_s32"
  BSW_VBrakeDigitalValue/1 -> Terminator4/1
  [GainParam] -> Bus Selector5/1
  [GainParam] -> Bus Selector7/1
  Minus1/1 -> Product1/1
  Bus Selector5/1 -> Product2/2  "<IGBTTempGain>"
  Product1/1 -> Data Type Conversion2/1
  [GainParam] -> Bus Selector3/1
  [OffsetParam] -> Bus Selector1/1
  Product3/1 -> Saturation/1
  Direct Lookup Table (n-D)2/1 -> MotorTemp1Value/1  "M_ADC_MotorTemp1Value_i16"
  Constant/1 -> Switch/1
  Compare To Constant/1 -> Switch/2
  Data Type Conversion2/1 -> Direct Lookup Table (n-D)2/1
  Direct Lookup Table (n-D)1/1 -> IGBTTempValue/1  "M_ADC_IGBTTempValue_i16"
  Product4/1 -> SMOUdcPuBase/1  "M_ADC_SMOUdcPuBase_s32"
  Product/1 -> Switch/3, Compare To Constant/1
  Bus Selector7/1 -> Product3/2  "<Acc1Gain>"
  Minus/1 -> Product/1
  BSW_IdcDigitalValue/1 -> Terminator6/1
  Minus3/1 -> Product3/1
  [OffsetParam] -> Bus Selector2/1
  Bus Selector3/1 -> Product1/2  "<MotorTempGain>"
  OffsetInit/1(OffsetParam) -> [OffsetParam]
  Product2/1 -> Data Type Conversion1/1
  BSW_VKeyDigitalValue/1 -> Terminator5/1
  [OffsetParam] -> Bus Selector6/1
  Bus Selector2/1 -> Minus1/2  "<MotorTemp1Offset>"
  BSW_HSTempDigitalValue/1 -> Terminator/1
  Bus Selector4/1 -> Minus2/2  "<IGBTTempOffset>"

== system MCU_Input/Input_10ms/GPIO_Get_10ms ==
  Compare To Constant : simulink/Logic and Bit Operations/Compare To Constant  relop===  const=ANALOG  OutDataTypeStr=boolean
  Constant : Constant  Value=ParamCfg_CommandSource_u16
  Read : Subsystem  TreatAsAtomicUnit=on
  Gpio_AntiTheftSignal : Outport
  Gpio_RepairSignal : Outport  Port=2
  Gpio_ABSSignal : Outport  Port=3
  Gpio_HDCSignal : Outport  Port=4
  Gpio_BackSignal : Outport  Port=5
  Gpio_CCSSignal : Outport  Port=6
  Gpio_SportSignal : Outport  Port=7
  Gpio_KGearSignal : Outport  Port=8
  Gpio_BrakeSignal : Outport  Port=9
  wires:
  Constant/1 -> Compare To Constant/1
  Compare To Constant/1 -> Read/Enable
  Read/1(Gpio_AntiTheftSignal) -> Gpio_AntiTheftSignal/1
  Read/3(Gpio_ABSSignal) -> Gpio_ABSSignal/1
  Read/2(Gpio_RepairSignal) -> Gpio_RepairSignal/1
  Read/4(Gpio_HDCSignal) -> Gpio_HDCSignal/1
  Read/5(Gpio_BackSignal) -> Gpio_BackSignal/1
  Read/6(Gpio_CCSSignal) -> Gpio_CCSSignal/1
  Read/7(Gpio_SportSignal) -> Gpio_SportSignal/1
  Read/8(Gpio_KGearSignal) -> Gpio_KGearSignal/1
  Read/9(Gpio_BrakeSignal) -> Gpio_BrakeSignal/1

== system MCU_Input/Input_10ms/低通滤波(并行) ==
  note: 母线电压的截止频率
  In1 : Inport
  Out1 : Outport
  wires:
  In1/1 -> Out1/1
